simulink model "VTOL_sim"  (R2018a)
settings: Solver=ode45  StartTime=0.0  StopTime=50  RelTol=1e-3  EnableMultiTasking=on
InitFcn:
  | addpath ./..
  | arm_param
  | armParamHW7
undefined symbols (not defined in the file or in its folder): P
settings Model: Creator=beard  LastModifiedBy=sadam
settings DataIOCC: LimitDataPoints=on  SaveFormat=Array  SignalLoggingSaveFormat=ModelDataLogs
settings OptimizationCC: ExpressionDepthLimit=2147483647  InitFltsAndDblsToZero=on  LifeSpan=inf
settings DebuggingCC: UnderspecifiedInitializationDetection=Classic  MergeDetectMultiDrivingBlocksExec=none  SolverPrmCheckMsg=warning  FcnCallInpInsideContextMsg=warning  StateNameClashWarn=warning  SFUnexpectedBacktrackingDiag=warning  SFNoUnconditionalDefaultTransitionDiag=warning  SFExecutionAtInitializationDiag=none
settings HardwareCC: ProdBitPerPointer=32  ProdBitPerSizeT=32  ProdBitPerPtrDiffT=32  ProdLargestAtomicFloat=None  ProdIntDivRoundTo=Undefined  ProdEndianess=Unspecified  ProdWordSize=32  ProdHWDeviceType=32-bit Generic
settings ModelReferenceCC: PropagateSignalLabelsOutOfModel=off
settings CodeAppCC: StateflowObjectComments=on
settings GRTTargetCC: TargetLangStandard=C89/C90 (ANSI)  GeneratePreprocessorConditionals=Disable all  CombineOutputUpdateFcns=off  GRTInterface=on
settings ConfigComp: CovMetricSettings=dw  CovHtmlReporting=on  CovSaveCumulativeToWorkspaceVar=on  CovSaveSingleToWorkspaceVar=on  CovExternalEMLEnable=off

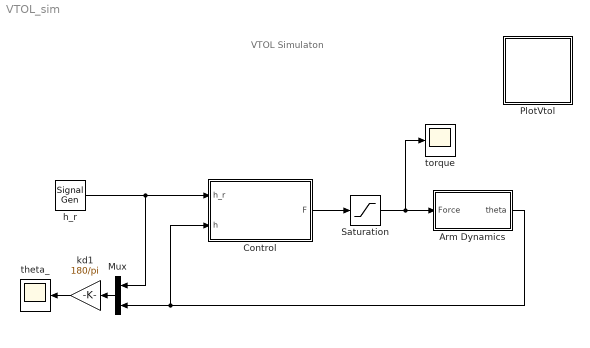
== system VTOL_sim ==
  note: VTOL Simulaton
  "Arm Dynamics " : Subsystem
  Control : Subsystem
  Mux : Mux  Inputs=2
  PlotVtol : Subsystem
      mask Display: image(imread('tv.jpg'))
  Saturation : Saturate  UpperLimit=P.Force_max  LowerLimit=-P.Force_max
  h_r : SignalGenerator  WaveForm=square  Amplitude=25*pi/180  Frequency=.05
  kd1 : Gain  Gain=180/pi
  theta_ : Scope
  torque : Scope
  wires:
  h_r/1 -> Control/1(h_r), Mux/1
  Mux/1 -> kd1/1
  kd1/1 -> theta_/1
  Control/1(F) -> Saturation/1
  Saturation/1 -> torque/1, "Arm Dynamics "/1(Force)
  "Arm Dynamics "/1("theta ") -> Control/2(h), Mux/2

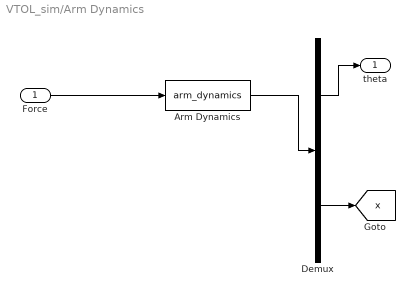
== system VTOL_sim/Arm Dynamics  ==
  Force : Inport
  Arm Dynamics : S-Function  FunctionName=arm_dynamics  Parameters=P  SFunctionDeploymentMode=off  EnableBusSupport=off
  Demux : Demux  Outputs=[1;2]
  "theta " : Outport
  tag scope: x=global
  wires:
  Force/1 -> Arm Dynamics/1
  Demux/1 -> "theta "/1
  Demux/2 -> [x]
  Arm Dynamics/1 -> Demux/1

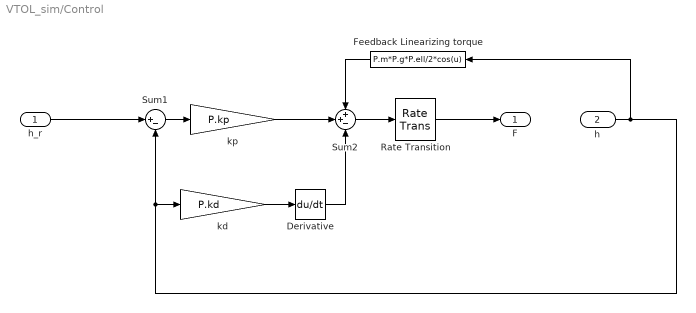
== system VTOL_sim/Control ==
  h_r : Inport
  h : Inport  Port=2
  Derivative : Derivative  CoefficientInTFapproximation=P.sigma
  Feedback Linearizing torque : Fcn  Expr=P.m*P.g*P.ell/2*cos(u)
  Rate Transition : RateTransition  OutPortSampleTime=P.Ts
  Sum1 : Sum  Inputs=|+-
  Sum2 : Sum  Inputs=++-
  kd : Gain  Gain=P.kd
  kp : Gain  Gain=P.kp
  F : Outport
  wires:
  Rate Transition/1 -> F/1
  h_r/1 -> Sum1/1
  Sum2/1 -> Rate Transition/1
  Sum1/1 -> kp/1
  kp/1 -> Sum2/2
  kd/1 -> Derivative/1
  Derivative/1 -> Sum2/3
  Feedback Linearizing torque/1 -> Sum2/1
  h/1 -> Feedback Linearizing torque/1, kd/1, Sum1/2

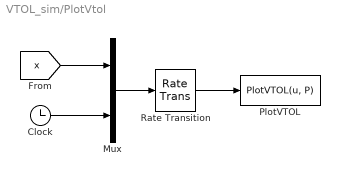
== system VTOL_sim/PlotVtol ==
  Clock : Clock
  Mux : Mux  Inputs=2
  "PlotVTOL " : MATLABFcn  MATLABFcn=PlotVTOL(u, P)  OutputDimensions=0
  Rate Transition : RateTransition  OutPortSampleTime=P.t_plot
  wires:
  Rate Transition/1 -> "PlotVTOL "/1
  Mux/1 -> Rate Transition/1
  Clock/1 -> Mux/2
  [x] -> Mux/1
